simulink model "SolarHeatSystemSimulation"  (R2023b)
settings: Solver=VariableStepAuto  StartTime=0.0  StopTime=1800  RelTol=1e-3
model workspace (MAT data in the model file):
  T_env = 293
  T_in = 288
  T_wi = 288
  cd_water = 4180
  density = 1000
  irradiance = 1000
  vol_flow = 0.0166666666667
libraries: simulink x1
settings Model: Creator=20241482  LastModifiedBy=20241482

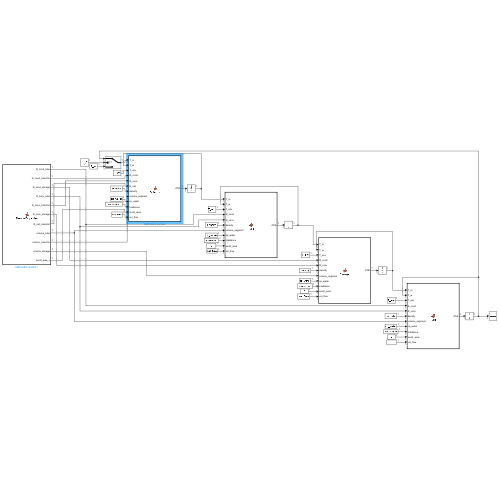
[thumbnail: Simulink's stored preview of the top-level diagram]
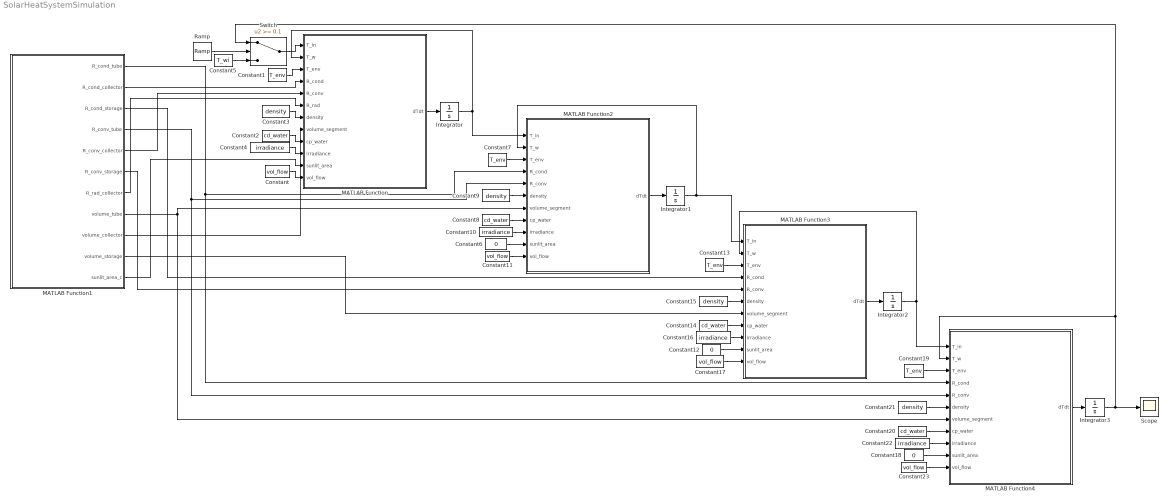
== system SolarHeatSystemSimulation ==
  Constant{,11,17,23} (4 alike) : Constant  Value=vol_flow
  Constant{1,7,13,19} (4 alike) : Constant  Value=T_env
  Constant{4,10,16,22} (4 alike) : Constant  Value=irradiance
  Constant12 : Constant  Value=0
  Constant{2,8,14,20} (4 alike) : Constant  Value=cd_water
  Constant{3,9,15,21} (4 alike) : Constant  Value=density
  Constant18 : Constant  Value=0
  Constant5 : Constant  Value=T_wi
  Constant6 : Constant  Value=0
  Integrator{,1..3} (4 alike) : Integrator  InitialCondition=288
  MATLAB Function : MATLAB Function  TreatAsAtomicUnit=on
  MATLAB Function1 : MATLAB Function  TreatAsAtomicUnit=on
  MATLAB Function2 : MATLAB Function  TreatAsAtomicUnit=on
  MATLAB Function3 : MATLAB Function  TreatAsAtomicUnit=on
  MATLAB Function4 : MATLAB Function  TreatAsAtomicUnit=on
  Ramp : simulink/Sources/Ramp  slope=1  start=0  InitialOutput=0
  Scope : Scope
  Switch : Switch  Threshold=0.1  SaturateOnIntegerOverflow=off  InputSameDT=off
  wires:
  MATLAB Function1/2(R_cond_collector) -> MATLAB Function/4(R_cond)
  MATLAB Function1/5(R_conv_collector) -> MATLAB Function/5(R_conv)
  Constant1/1 -> MATLAB Function/3(T_env)
  Constant2/1 -> MATLAB Function/9(cp_water)
  Constant3/1 -> MATLAB Function/7(density)
  Constant4/1 -> MATLAB Function/10(irradiance)
  MATLAB Function1/9(volume_collector) -> MATLAB Function/8(volume_segment)
  Constant7/1 -> MATLAB Function2/3(T_env)
  Constant6/1 -> MATLAB Function2/10(sunlit_area)
  Constant10/1 -> MATLAB Function2/9(irradiance)
  Constant9/1 -> MATLAB Function2/6(density)
  Constant13/1 -> MATLAB Function3/3(T_env)
  Constant12/1 -> MATLAB Function3/10(sunlit_area)
  Constant16/1 -> MATLAB Function3/9(irradiance)
  Constant15/1 -> MATLAB Function3/6(density)
  Constant19/1 -> MATLAB Function4/3(T_env)
  Constant18/1 -> MATLAB Function4/10(sunlit_area)
  Constant22/1 -> MATLAB Function4/9(irradiance)
  Constant21/1 -> MATLAB Function4/6(density)
  MATLAB Function1/11(sunlit_area_c) -> MATLAB Function/11(sunlit_area)
  MATLAB Function1/3(R_cond_storage) -> MATLAB Function3/4(R_cond)
  MATLAB Function1/6(R_conv_storage) -> MATLAB Function3/5(R_conv)
  MATLAB Function1/10(volume_storage) -> MATLAB Function3/7(volume_segment)
  MATLAB Function1/1(R_cond_tube) -> MATLAB Function4/4(R_cond), MATLAB Function2/4(R_cond)
  MATLAB Function1/4(R_conv_tube) -> MATLAB Function4/5(R_conv), MATLAB Function2/5(R_conv)
  MATLAB Function1/8(volume_tube) -> MATLAB Function2/7(volume_segment), MATLAB Function4/7(volume_segment)
  Constant5/1 -> Switch/3
  Switch/1 -> MATLAB Function/1(T_in)
  Constant8/1 -> MATLAB Function2/8(cp_water)
  Constant14/1 -> MATLAB Function3/8(cp_water)
  Constant20/1 -> MATLAB Function4/8(cp_water)
  Constant/1 -> MATLAB Function/12(vol_flow)
  Constant11/1 -> MATLAB Function2/11(vol_flow)
  Constant17/1 -> MATLAB Function3/11(vol_flow)
  Constant23/1 -> MATLAB Function4/11(vol_flow)
  MATLAB Function/1(dTdt) -> Integrator/1
  Integrator/1 -> MATLAB Function2/1(T_in), MATLAB Function/2(T_w)
  MATLAB Function2/1(dTdt) -> Integrator1/1
  Integrator1/1 -> MATLAB Function3/1(T_in), MATLAB Function2/2(T_w)
  MATLAB Function3/1(dTdt) -> Integrator2/1
  Integrator2/1 -> MATLAB Function3/2(T_w), MATLAB Function4/1(T_in)
  Integrator3/1 -> Scope/1, Switch/1, MATLAB Function4/2(T_w)
  MATLAB Function4/1(dTdt) -> Integrator3/1
  Ramp/1 -> Switch/2
  MATLAB Function1/7(R_rad_collector) -> MATLAB Function/6(R_rad)

== matlab function SolarHeatSystemSimulation/MATLAB Function1 ==
  data: R_cond_tube output; R_cond_collector output; R_cond_storage output; R_conv_tube output; R_conv_collector output; R_conv_storage output; R_rad_collector output; volume_tube output; volume_collector output; volume_storage output; sunlit_area_c output
function [R_cond_tube, R_cond_collector, R_cond_storage, R_conv_tube, R_conv_collector, R_conv_storage, R_rad_collector, volume_tube, volume_collector, volume_storage, sunlit_area_c] = ThermalProperties()

S_B = 5.67*10e-9; % Stefan-Boltzmann
h_c_air = 25.5; % Natural convection, 25-20 C, 1 atm

k_pvc = 0.19;
k_i = 0.022;
k_floor = 0.30;
k_al = 237;
k_PU = 0.13;

em_pvc = 0.92;
em_i = 0.8;     % Approximate values based on color
em_floor = 0.1; % and intuition. Exact values
em_PU = 0.9;    % could not be found on the Internet.

d_in = 0.0085;
d_out = 0.012;
L = 1;
R_cond_tube = log(d_out/d_in)/(2*pi*k_PU*L);
R_conv_tube = 1/(h_c_air*2*pi*(d_out/2)*L);
R_rad_tube = 1/(S_B*2*pi*em_PU*(d_out/2)*L);
volume_tube = pi*L*(d_in/2)^2;

d_c = 0.001;     % Not mentioned
d_al = 0.002;    %
d_table = 0.006;
A_c = 1.44;
R_cond_collector = 1/(1/(d_c/(A_c*k_pvc))+1/((d_c/(A_c*k_pvc))+(d_al/(A_c*k_al))+(d_table/(A_c*k_floor))));
R_conv_collector = 1/(2*h_c_air*A_c);
R_rad_collector = 1/(S_B*A_c*(em_floor+em_pvc));
volume_collector = 0.005; % Max volume is about 10 liters. Assuming half full to not waste water.
sunlit_area_c = A_c;

D_t = 0.11;
d_wall = 0.002; % Not mentioned
d_i = 0.02;
d_lid = 0.005;  %
d_floor = 0.01; %
d_tube = d_out;
H = 0.2;
A_floor = pi*(D_t/2)^2;
A_lid = A_floor - 2*pi*(d_tube/2)^2;
R_cond_storage = 1/(1/(log((D_t/2+d_wall)/(D_t/2))/(2*pi*k_pvc*H)+log((D_t/2+d_wall+d_i)/(D_t/2+d_wall))/(2*pi*k_i*H))+1/((d_wall/(A_floor*k_pvc))+(d_i/(A_floor*k_i))+(d_floor/(A_floor*k_floor)))+1/(d_lid/(A_lid*k_pvc)));
R_conv_storage = 1/((h_c_air*2*pi*((D_t/2+d_wall+d_i)/2)*H)+(h_c_air*2*pi*A_floor)+(h_c_air*2*pi*A_lid));
R_rad_storage = 1/((S_B*2*pi*em_i*((D_t/2+d_wall+d_i)/2)*H)+(S_B*2*pi*em_floor*A_floor)+(S_B*2*pi*em_pvc*A_lid));
volume_storage = 0.002;

== matlab function SolarHeatSystemSimulation/MATLAB Function ==
  data: T_in input; T_w input; dTdt output; T_env input; R_cond input; R_conv input; R_rad input; density input; volume_segment input; cp_water input; irradiance input; sunlit_area input; vol_flow input
function dTdt  = Collector (T_in, T_w, T_env, R_cond, R_conv, R_rad, density, volume_segment, cp_water, irradiance, sunlit_area, vol_flow)

    a = [1/R_rad, 0, 0, (1/R_cond + 1/R_conv), -(irradiance*sunlit_area + (T_env^4)/R_rad + T_w/R_cond + T_env/R_conv)];

    Ts = roots(a);

    for i = 1:4
        if isreal(Ts(i)) == true && Ts(i) > 0 
            T_outer = Ts(i);
        end
    end

    %T_outer = ((irradiance*sunlit_area)+T_w/R_cond+T_env/R_conv)/(1/R_cond + 1/R_conv);

    Q_dot = density*vol_flow*cp_water*(T_in-T_w) - (T_w - T_outer)/R_cond; % solve for heat conducted from water to outer surface

    dTdt = Q_dot / (density * volume_segment * cp_water); % change in temperature over segment
end

== matlab function SolarHeatSystemSimulation/MATLAB Function2 ==
  data: T_in input; T_w input; dTdt output; T_env input; R_cond input; R_conv input; density input; volume_segment input; cp_water input; irradiance input; sunlit_area input; vol_flow input
function dTdt  = Tube (T_in, T_w, T_env, R_cond, R_conv, density, volume_segment, cp_water, irradiance, sunlit_area, vol_flow)

    T_outer = ((irradiance*sunlit_area)+T_w/R_cond+T_env/R_conv)/(1/R_cond + 1/R_conv);

    Q_dot = density*vol_flow*cp_water*(T_in-T_w) - (T_w - T_outer)/R_cond; % solve for heat conducted from water to outer surface

    dTdt = Q_dot / (density * volume_segment * cp_water); % change in temperature over segment

end

== matlab function SolarHeatSystemSimulation/MATLAB Function3 ==
  data: T_in input; T_w input; dTdt output; T_env input; R_cond input; R_conv input; density input; volume_segment input; cp_water input; irradiance input; sunlit_area input; vol_flow input
function dTdt  = Storage (T_in, T_w, T_env, R_cond, R_conv, density, volume_segment, cp_water, irradiance, sunlit_area, vol_flow)

    T_outer = ((irradiance*sunlit_area)+T_w/R_cond+T_env/R_conv)/(1/R_cond + 1/R_conv);

    Q_dot = density*vol_flow*cp_water*(T_in-T_w) - (T_w - T_outer)/R_cond; % solve for heat conducted from water to outer surface

    dTdt = Q_dot / (density * volume_segment * cp_water); % change in temperature over segment
end

== matlab function SolarHeatSystemSimulation/MATLAB Function4 ==
  data: T_in input; T_w input; dTdt output; T_env input; R_cond input; R_conv input; density input; volume_segment input; cp_water input; irradiance input; sunlit_area input; vol_flow input
function dTdt  = Tube (T_in, T_w, T_env, R_cond, R_conv, density, volume_segment, cp_water, irradiance, sunlit_area, vol_flow)

    T_outer = ((irradiance*sunlit_area)+T_w/R_cond+T_env/R_conv)/(1/R_cond + 1/R_conv);

    Q_dot = density*vol_flow*cp_water*(T_in-T_w) - (T_w - T_outer)/R_cond; % solve for heat conducted from water to outer surface

    dTdt = Q_dot / (density * volume_segment * cp_water); % change in temperature over segment

end
